simulink library "PRISMA"  (R2025b)
settings: Solver=VariableStepAuto  StartTime=0.0  StopTime=10.0  RelTol=1e-3
libraries: $bdroot x116, etargetslib x30, simulink x9
(part 3 of 3)

== system PRISMA/Transformation/Transform Quaternion OpenGL to NED ==
  OpenGL : Inport  OutDataTypeStr=double  PortDimensions=4
  Mux : Mux
  Selector : Selector  InputPortWidth=4  IndexOptions=Index vector (dialog)  Indices=3  OutputSizes=1
  Selector1 : Selector  InputPortWidth=4  IndexOptions=Index vector (dialog)  Indices=2  OutputSizes=1
  Selector2 : Selector  InputPortWidth=4  IndexOptions=Index vector (dialog)  Indices=4  OutputSizes=1
  Selector3 : Selector  InputPortWidth=4  IndexOptions=Index vector (dialog)  Indices=1  OutputSizes=1
  Unary Minus : UnaryMinus
  Unary Minus1 : UnaryMinus
  NED : Outport  OutDataTypeStr=double  PortDimensions=4
  wires:
  Selector3/1 -> Mux/1
  OpenGL/1 -> Selector/1, Selector1/1, Selector2/1, Selector3/1
  Mux/1 -> NED/1
  Unary Minus/1 -> Mux/2
  Unary Minus1/1 -> Mux/4
  Selector2/1 -> Unary Minus/1
  Selector1/1 -> Mux/3
  Selector/1 -> Unary Minus1/1

== system PRISMA/Transformation/Transform Scale NED to OpenGL ==
  NED : Inport  OutDataTypeStr=double  PortDimensions=3
  Mux : Mux  Inputs=3
  Selector : Selector  InputPortWidth=3  IndexOptions=Index vector (dialog)  Indices=2  OutputSizes=1
  Selector1 : Selector  InputPortWidth=3  IndexOptions=Index vector (dialog)  Indices=1  OutputSizes=1
  Selector2 : Selector  InputPortWidth=3  IndexOptions=Index vector (dialog)  Indices=3  OutputSizes=1
  OpenGL : Outport  OutDataTypeStr=double  PortDimensions=3
  wires:
  Mux/1 -> OpenGL/1
  NED/1 -> Selector2/1, Selector1/1, Selector/1
  Selector2/1 -> Mux/2
  Selector/1 -> Mux/1
  Selector1/1 -> Mux/3

== system PRISMA/Transformation/Transform Scale OpenGL to NED ==
  OpenGL : Inport  OutDataTypeStr=double  PortDimensions=3
  Mux : Mux  Inputs=3
  Selector : Selector  InputPortWidth=3  IndexOptions=Index vector (dialog)  Indices=3  OutputSizes=1
  Selector1 : Selector  InputPortWidth=3  IndexOptions=Index vector (dialog)  Indices=2  OutputSizes=1
  Selector2 : Selector  InputPortWidth=3  IndexOptions=Index vector (dialog)  Indices=1  OutputSizes=1
  NED : Outport  OutDataTypeStr=double  PortDimensions=3
  wires:
  Selector1/1 -> Mux/3
  OpenGL/1 -> Selector2/1, Selector1/1, Selector/1
  Selector2/1 -> Mux/2
  Mux/1 -> NED/1
  Selector/1 -> Mux/1

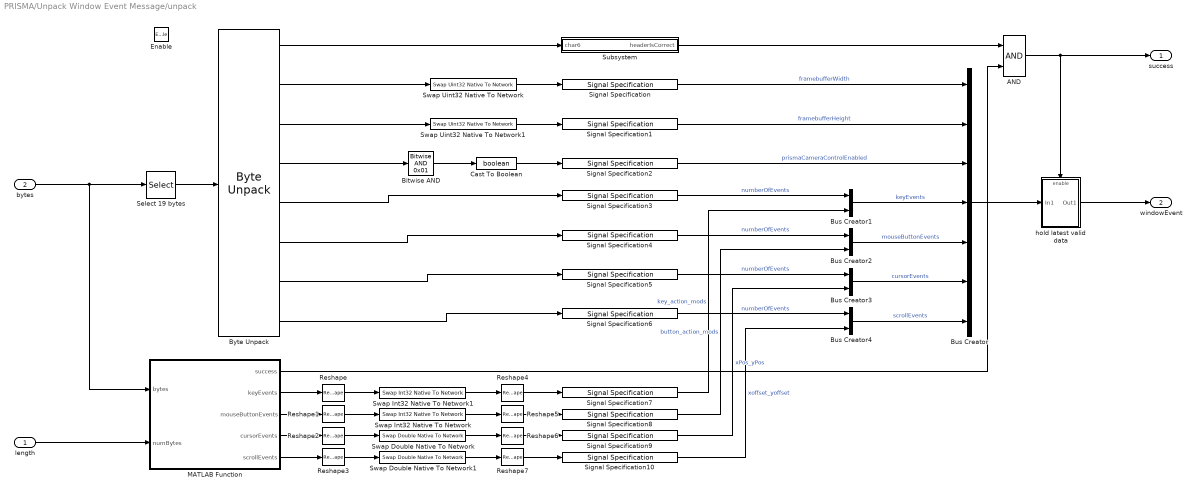
== system PRISMA/Unpack Window Event Message/unpack ==
  length : Inport
  bytes : Inport  Port=2
  Enable : EnablePort
  AND : Logic  AllPortsSameDT=off  OutDataTypeStr=boolean
  Bitwise AND : simulink/Logic and Bit Operations/Bitwise Operator  logicop=AND  UseBitMask=on  BitMask=0x01  BitMaskRealWorld=Stored Integer
      settings: LibrarySourceBlock=|
      | simulink/Quick Insert/Logic and Bit
      | Operations/Bitwise AND
  Bus Creator : BusCreator  Inputs=7
  Bus Creator{1..4} (4 alike) : BusCreator  Inputs=2
  Byte Unpack : etargetslib/Byte Unpack  dimensions={6,1,1,1,1,1,1,1}  datatypes={'uint8','uint32','uint32','uint8','uint8','uint8','uint8','uint8'}  byteAlign=1
      settings: LibrarySourceBlock=embeddedtargetslib/Host Communication/Byte Unpack
  Cast To Boolean : DataTypeConversion  OutDataTypeStr=boolean  SaturateOnIntegerOverflow=off  RndMeth=Floor
  MATLAB Function : MATLAB Function  TreatAsAtomicUnit=on
  Reshape{,1..3} (4 alike) : Reshape
  Reshape4 : Reshape  OutputDimensionality=Customize  OutputDimensions=[255,3]
  Reshape5 : Reshape  OutputDimensionality=Customize  OutputDimensions=[255,3]
  Reshape6 : Reshape  OutputDimensionality=Customize  OutputDimensions=[255,2]
  Reshape7 : Reshape  OutputDimensionality=Customize  OutputDimensions=[255,2]
  Select 19 bytes : Selector  IndexOptions=Index vector (dialog)  Indices=1:19  OutputSizes=1
  Signal Specification : SignalSpecification  OutDataTypeStr=uint32  Dimensions=1
  Signal Specification1 : SignalSpecification  OutDataTypeStr=uint32  Dimensions=1
  Signal Specification10 : SignalSpecification  OutDataTypeStr=double  Dimensions=[255,2]
  Signal Specification2 : SignalSpecification  OutDataTypeStr=boolean  Dimensions=1
  Signal Specification{3..6} (4 alike) : SignalSpecification  OutDataTypeStr=uint8  Dimensions=1
  Signal Specification7 : SignalSpecification  OutDataTypeStr=int32  Dimensions=[255,3]
  Signal Specification8 : SignalSpecification  OutDataTypeStr=int32  Dimensions=[255,3]
  Signal Specification9 : SignalSpecification  OutDataTypeStr=double  Dimensions=[255,2]
  Subsystem : Subsystem
  Swap Double Native To Network : $bdroot/details/Swap Double Native To Network
  Swap Double Native To Network1 : $bdroot/details/Swap Double Native To Network
  Swap Int32 Native To Network : $bdroot/details/Swap Int32 Native To Network
  Swap Int32 Native To Network1 : $bdroot/details/Swap Int32 Native To Network
  Swap Uint32 Native To Network : $bdroot/details/Swap Uint32 Native To Network
  Swap Uint32 Native To Network1 : $bdroot/details/Swap Uint32 Native To Network
  hold latest valid data : Subsystem  TreatAsAtomicUnit=on
  success : Outport  OutDataTypeStr=boolean  PortDimensions=1
  windowEvent : Outport  Port=2
  wires:
  Cast To Boolean/1 -> Signal Specification2/1
  Select 19 bytes/1 -> Byte Unpack/1
  bytes/1 -> Select 19 bytes/1, MATLAB Function/1(bytes)
  Byte Unpack/2 -> Swap Uint32 Native To Network/1
  Byte Unpack/3 -> Swap Uint32 Native To Network1/1
  Byte Unpack/1 -> Subsystem/1(char6)
  Signal Specification/1 -> Bus Creator/1  "framebufferWidth"
  Signal Specification1/1 -> Bus Creator/2  "framebufferHeight"
  Byte Unpack/4 -> Bitwise AND/1
  Bitwise AND/1 -> Cast To Boolean/1
  Byte Unpack/5 -> Signal Specification3/1
  Byte Unpack/6 -> Signal Specification4/1
  Byte Unpack/7 -> Signal Specification5/1
  Byte Unpack/8 -> Signal Specification6/1
  Signal Specification2/1 -> Bus Creator/3  "prismaCameraControlEnabled"
  length/1 -> MATLAB Function/2(numBytes)
  MATLAB Function/2(keyEvents) -> Reshape/1
  MATLAB Function/3(mouseButtonEvents) -> Reshape1/1
  Signal Specification7/1 -> Bus Creator1/2  "key_action_mods"
  Signal Specification8/1 -> Bus Creator2/2  "button_action_mods"
  MATLAB Function/4(cursorEvents) -> Reshape2/1
  MATLAB Function/5(scrollEvents) -> Reshape3/1
  Signal Specification9/1 -> Bus Creator3/2  "xPos_yPos"
  Signal Specification10/1 -> Bus Creator4/2  "xoffset_yoffset"
  Signal Specification3/1 -> Bus Creator1/1  "numberOfEvents"
  Bus Creator1/1 -> Bus Creator/4  "keyEvents"
  Bus Creator2/1 -> Bus Creator/5  "mouseButtonEvents"
  Signal Specification4/1 -> Bus Creator2/1  "numberOfEvents"
  Bus Creator3/1 -> Bus Creator/6  "cursorEvents"
  Signal Specification5/1 -> Bus Creator3/1  "numberOfEvents"
  Bus Creator4/1 -> Bus Creator/7  "scrollEvents"
  Signal Specification6/1 -> Bus Creator4/1  "numberOfEvents"
  Subsystem/1(headerIsCorrect) -> AND/1
  MATLAB Function/1(success) -> AND/2
  AND/1 -> success/1, hold latest valid data/Enable
  Bus Creator/1 -> hold latest valid data/1(In1)
  hold latest valid data/1(Out1) -> windowEvent/1
  Swap Uint32 Native To Network/1 -> Signal Specification/1
  Swap Uint32 Native To Network1/1 -> Signal Specification1/1
  Swap Double Native To Network/1 -> Reshape6/1
  Swap Double Native To Network1/1 -> Reshape7/1
  Swap Int32 Native To Network/1 -> Reshape5/1
  Swap Int32 Native To Network1/1 -> Reshape4/1
  Reshape/1 -> Swap Int32 Native To Network1/1
  Reshape1/1 -> Swap Int32 Native To Network/1
  Reshape2/1 -> Swap Double Native To Network/1
  Reshape3/1 -> Swap Double Native To Network1/1
  Reshape4/1 -> Signal Specification7/1
  Reshape5/1 -> Signal Specification8/1
  Reshape6/1 -> Signal Specification9/1
  Reshape7/1 -> Signal Specification10/1

== system PRISMA/details/PRISMA Bitfield To Byte ==
  bitfield : Inport  OutDataTypeStr=boolean  PortDimensions=8
  Bitwise Operator : simulink/Logic and Bit Operations/Bitwise Operator  logicop=OR  UseBitMask=off  NumInputPorts=8  BitMask=bin2dec('11011001')  BitMaskRealWorld=Stored Integer
  Data Type Conversion : DataTypeConversion  OutDataTypeStr=uint8  SaturateOnIntegerOverflow=off  RndMeth=Floor
  Demux6 : Demux  Outputs=8
  Shift Arithmetic : ArithShift  BitShiftNumber=1  BitShiftDirection=Left
  Shift Arithmetic1 : ArithShift  BitShiftNumber=2  BitShiftDirection=Left
  Shift Arithmetic2 : ArithShift  BitShiftNumber=3  BitShiftDirection=Left
  Shift Arithmetic3 : ArithShift  BitShiftNumber=4  BitShiftDirection=Left
  Shift Arithmetic4 : ArithShift  BitShiftNumber=5  BitShiftDirection=Left
  Shift Arithmetic5 : ArithShift  BitShiftNumber=6  BitShiftDirection=Left
  Shift Arithmetic6 : ArithShift  BitShiftNumber=7  BitShiftDirection=Left
  byte : Outport  OutDataTypeStr=uint8  PortDimensions=1
  wires:
  Demux6/4 -> Shift Arithmetic2/1
  Demux6/5 -> Shift Arithmetic3/1
  Data Type Conversion/1 -> Demux6/1
  Demux6/2 -> Shift Arithmetic/1
  Shift Arithmetic1/1 -> Bitwise Operator/3
  Demux6/7 -> Shift Arithmetic5/1
  Demux6/6 -> Shift Arithmetic4/1
  Shift Arithmetic6/1 -> Bitwise Operator/8
  Shift Arithmetic5/1 -> Bitwise Operator/7
  Shift Arithmetic/1 -> Bitwise Operator/2
  Demux6/1 -> Bitwise Operator/1
  Demux6/3 -> Shift Arithmetic1/1
  Shift Arithmetic4/1 -> Bitwise Operator/6
  Demux6/8 -> Shift Arithmetic6/1
  Bitwise Operator/1 -> byte/1
  Shift Arithmetic3/1 -> Bitwise Operator/5
  Shift Arithmetic2/1 -> Bitwise Operator/4
  bitfield/1 -> Data Type Conversion/1

== system PRISMA/details/PRISMA Message Type ==
  value : Constant  Value=messageType - 1  OutDataTypeStr=uint8
  byte : Outport  OutDataTypeStr=uint8  PortDimensions=1
  wires:
  value/1 -> byte/1

== system PRISMA/details/Swap Double Native To Network ==
  note: Check endianess of this machine
      | (only swap on little-endian-based machines)
  in : Inport  OutDataTypeStr=double
  Byte Pack1 : etargetslib/Byte Pack  datatypes={'uint16'}  byteAlign=1
  Constant : Constant  Value=uint16(1)
  Selector2 : Selector  InputPortWidth=2  IndexOptions=Index vector (dialog)  Indices=1  OutputSizes=1
  Swap Each Element : Subsystem  TreatAsAtomicUnit=on
  Switch : Switch  Criteria=u2 ~= 0  SaturateOnIntegerOverflow=off  InputSameDT=off
  out : Outport  OutDataTypeStr=double
  wires:
  Switch/1 -> out/1
  Selector2/1 -> Switch/2
  Swap Each Element/1(out) -> Switch/1
  Byte Pack1/1 -> Selector2/1
  in/1 -> Swap Each Element/1(in), Switch/3
  Constant/1 -> Byte Pack1/1

== system PRISMA/details/Swap Float Native To Network ==
  note: Check endianess of this machine
      | (only swap on little-endian-based machines)
  in : Inport  OutDataTypeStr=single
  Byte Pack1 : etargetslib/Byte Pack  datatypes={'uint16'}  byteAlign=1
  Constant : Constant  Value=uint16(1)
  Selector2 : Selector  InputPortWidth=2  IndexOptions=Index vector (dialog)  Indices=1  OutputSizes=1
  Swap Each Element : Subsystem  TreatAsAtomicUnit=on
  Switch : Switch  Criteria=u2 ~= 0  SaturateOnIntegerOverflow=off  InputSameDT=off
  out : Outport  OutDataTypeStr=single
  wires:
  Constant/1 -> Byte Pack1/1
  in/1 -> Switch/3, Swap Each Element/1(in)
  Byte Pack1/1 -> Selector2/1
  Swap Each Element/1(out) -> Switch/1
  Selector2/1 -> Switch/2
  Switch/1 -> out/1

== system PRISMA/details/Swap Int32 Native To Network ==
  note: Check endianess of this machine
      | (only swap on little-endian-based machines)
  in : Inport  OutDataTypeStr=int32
  Byte Pack1 : etargetslib/Byte Pack  datatypes={'uint16'}  byteAlign=1
  Constant : Constant  Value=uint16(1)
  Selector2 : Selector  InputPortWidth=2  IndexOptions=Index vector (dialog)  Indices=1  OutputSizes=1
  Swap Each Element : Subsystem  TreatAsAtomicUnit=on
  Switch : Switch  Criteria=u2 ~= 0  SaturateOnIntegerOverflow=off  InputSameDT=off
  out : Outport  OutDataTypeStr=int32
  wires:
  Constant/1 -> Byte Pack1/1
  in/1 -> Switch/3, Swap Each Element/1(in)
  Byte Pack1/1 -> Selector2/1
  Swap Each Element/1(out) -> Switch/1
  Selector2/1 -> Switch/2
  Switch/1 -> out/1

== system PRISMA/details/Swap Uint16 Native To Network ==
  note: Check endianess of this machine
      | (only swap on little-endian-based machines)
  in : Inport  OutDataTypeStr=uint16
  Byte Pack1 : etargetslib/Byte Pack  datatypes={'uint16'}  byteAlign=1
  Constant : Constant  Value=uint16(1)
  Selector2 : Selector  InputPortWidth=2  IndexOptions=Index vector (dialog)  Indices=1  OutputSizes=1
  Swap Each Element : Subsystem  TreatAsAtomicUnit=on
  Switch : Switch  Criteria=u2 ~= 0  SaturateOnIntegerOverflow=off  InputSameDT=off
  out : Outport  OutDataTypeStr=uint16
  wires:
  Switch/1 -> out/1
  Selector2/1 -> Switch/2
  Swap Each Element/1(out) -> Switch/1
  Byte Pack1/1 -> Selector2/1
  in/1 -> Swap Each Element/1(in), Switch/3
  Constant/1 -> Byte Pack1/1

== system PRISMA/details/Swap Uint32 Native To Network ==
  note: Check endianess of this machine
      | (only swap on little-endian-based machines)
  in : Inport  OutDataTypeStr=uint32
  Byte Pack1 : etargetslib/Byte Pack  datatypes={'uint16'}  byteAlign=1
  Constant : Constant  Value=uint16(1)
  Selector2 : Selector  InputPortWidth=2  IndexOptions=Index vector (dialog)  Indices=1  OutputSizes=1
  Swap Each Element : Subsystem  TreatAsAtomicUnit=on
  Switch : Switch  Criteria=u2 ~= 0  SaturateOnIntegerOverflow=off  InputSameDT=off
  out : Outport  OutDataTypeStr=uint32
  wires:
  Switch/1 -> out/1
  Selector2/1 -> Switch/2
  Swap Each Element/1(out) -> Switch/1
  Byte Pack1/1 -> Selector2/1
  in/1 -> Swap Each Element/1(in), Switch/3
  Constant/1 -> Byte Pack1/1

== system PRISMA/Unpack Window Event Message/unpack/Subsystem ==
  char6 : Inport
  AND : Logic  Inputs=6  AllPortsSameDT=off  OutDataTypeStr=boolean
  Compare To Constant : simulink/Logic and Bit Operations/Compare To Constant  relop===  const=uint8('P')  OutDataTypeStr=boolean
  Compare To Constant1 : simulink/Logic and Bit Operations/Compare To Constant  relop===  const=uint8('R')  OutDataTypeStr=boolean
  Compare To Constant2 : simulink/Logic and Bit Operations/Compare To Constant  relop===  const=uint8('I')  OutDataTypeStr=boolean
  Compare To Constant3 : simulink/Logic and Bit Operations/Compare To Constant  relop===  const=uint8('S')  OutDataTypeStr=boolean
  Compare To Constant4 : simulink/Logic and Bit Operations/Compare To Constant  relop===  const=uint8('M')  OutDataTypeStr=boolean
  Compare To Constant5 : simulink/Logic and Bit Operations/Compare To Constant  relop===  const=uint8('A')  OutDataTypeStr=boolean
  Demux : Demux  Outputs=6
  headerIsCorrect : Outport
  wires:
  Demux/5 -> Compare To Constant4/1
  Compare To Constant1/1 -> AND/2
  Compare To Constant2/1 -> AND/3
  Demux/2 -> Compare To Constant1/1
  Compare To Constant5/1 -> AND/6
  Demux/1 -> Compare To Constant/1
  Demux/3 -> Compare To Constant2/1
  Demux/4 -> Compare To Constant3/1
  Compare To Constant3/1 -> AND/4
  Compare To Constant/1 -> AND/1
  Compare To Constant4/1 -> AND/5
  Demux/6 -> Compare To Constant5/1
  AND/1 -> headerIsCorrect/1
  char6/1 -> Demux/1

== system PRISMA/Unpack Window Event Message/unpack/hold latest valid data ==
  In1 : Inport
  Enable : EnablePort
  Out1 : Outport
  wires:
  In1/1 -> Out1/1

== system PRISMA/details/Swap Double Native To Network/Swap Each Element ==
  in : Inport  Partition=on  PartitionDimension=1  PartitionWidth=1  PartitionOffset=0
  Byte Pack : etargetslib/Byte Pack  datatypes={'double'}  byteAlign=1
  Byte Unpack : etargetslib/Byte Unpack  dimensions={[1]}  datatypes={'double'}  byteAlign=1
  For Each : ForEach  DisableCoverage=on
  Selector : Selector  InputPortWidth=8  IndexOptions=Index vector (dialog)  Indices=[8 7 6 5 4 3 2 1]  OutputSizes=1
  out : Outport  ConcatenationDimension=1
  wires:
  in/1 -> Byte Pack/1
  Byte Unpack/1 -> out/1
  Byte Pack/1 -> Selector/1
  Selector/1 -> Byte Unpack/1

== system PRISMA/details/Swap Float Native To Network/Swap Each Element ==
  in : Inport  Partition=on  PartitionDimension=1  PartitionWidth=1  PartitionOffset=0
  Byte Pack : etargetslib/Byte Pack  datatypes={'single'}  byteAlign=1
  Byte Unpack : etargetslib/Byte Unpack  dimensions={[1]}  datatypes={'single'}  byteAlign=1
  For Each : ForEach  DisableCoverage=on
  Selector : Selector  InputPortWidth=4  IndexOptions=Index vector (dialog)  Indices=[4 3 2 1]  OutputSizes=1
  out : Outport  ConcatenationDimension=1
  wires:
  Selector/1 -> Byte Unpack/1
  Byte Pack/1 -> Selector/1
  Byte Unpack/1 -> out/1
  in/1 -> Byte Pack/1

== system PRISMA/details/Swap Int32 Native To Network/Swap Each Element ==
  in : Inport  Partition=on  PartitionDimension=1  PartitionWidth=1  PartitionOffset=0
  Byte Pack : etargetslib/Byte Pack  datatypes={'int32'}  byteAlign=1
  Byte Unpack : etargetslib/Byte Unpack  dimensions={[1]}  datatypes={'int32'}  byteAlign=1
  For Each : ForEach  DisableCoverage=on
  Selector : Selector  InputPortWidth=4  IndexOptions=Index vector (dialog)  Indices=[4 3 2 1]  OutputSizes=1
  out : Outport  ConcatenationDimension=1
  wires:
  Selector/1 -> Byte Unpack/1
  Byte Pack/1 -> Selector/1
  Byte Unpack/1 -> out/1
  in/1 -> Byte Pack/1

== system PRISMA/details/Swap Uint16 Native To Network/Swap Each Element ==
  in : Inport  Partition=on  PartitionDimension=1  PartitionWidth=1  PartitionOffset=0
  Byte Pack : etargetslib/Byte Pack  datatypes={'uint16'}  byteAlign=1
  Byte Unpack : etargetslib/Byte Unpack  dimensions={[1]}  datatypes={'uint16'}  byteAlign=1
  For Each : ForEach  DisableCoverage=on
  Selector : Selector  InputPortWidth=2  IndexOptions=Index vector (dialog)  Indices=[2 1]  OutputSizes=1
  out : Outport  ConcatenationDimension=1
  wires:
  in/1 -> Byte Pack/1
  Byte Unpack/1 -> out/1
  Byte Pack/1 -> Selector/1
  Selector/1 -> Byte Unpack/1

== system PRISMA/details/Swap Uint32 Native To Network/Swap Each Element ==
  in : Inport  Partition=on  PartitionDimension=1  PartitionWidth=1  PartitionOffset=0
  Byte Pack : etargetslib/Byte Pack  datatypes={'uint32'}  byteAlign=1
  Byte Unpack : etargetslib/Byte Unpack  dimensions={[1]}  datatypes={'uint32'}  byteAlign=1
  For Each : ForEach  DisableCoverage=on
  Selector : Selector  InputPortWidth=4  IndexOptions=Index vector (dialog)  Indices=[4 3 2 1]  OutputSizes=1
  out : Outport  ConcatenationDimension=1
  wires:
  in/1 -> Byte Pack/1
  Byte Unpack/1 -> out/1
  Byte Pack/1 -> Selector/1
  Selector/1 -> Byte Unpack/1

== matlab function PRISMA/Transformation/Euler ZYX to Quaternion/MATLAB Function ==
  data: roll input; q output; pitch input; yaw input
function q = EulerToQuaternionZYX(roll, pitch, yaw)
    q = eul2quat([yaw, pitch, roll],'ZYX')';
end

== matlab function PRISMA/Pack Watermesh Message/Serialize To Network Byte Order ==
  data: vertexData input single size=[2,255,32]; bytes output uint8 size=65280; numVertices input uint8 size=32; numPolygons input uint8 size=1; numBytes output int32 size=1
function [bytes, numBytes] = SerializeWatermeshData(vertexData, numVertices, numPolygons)
    tmp = typecast(uint16(1),'uint8');
    swapByteOrder = (tmp(1) == uint8(1));

    % output size
    bytes = uint8(zeros(65280,1)); % 2*255*32 * 4
    numBytes = int32(0);

    % number of polygons (2 bytes)
    numPolygons = uint16(min(uint16(numPolygons), uint16(32)));
    bytes(1:2) = reshape(typecast(uint16(numPolygons),'uint8'), [2 1]);
    if(swapByteOrder)
        h = bytes(1);
        bytes(1) = bytes(2);
        bytes(2) = h;
    end

    % serialize all polygons
    index = int32(3);
    if(swapByteOrder)
        for p = uint32(1):uint32(numPolygons)
            % number of vertices (2 bytes)
            N = uint16(numVertices(p));
            bytes(index:(index+int32(1))) = reshape(typecast(uint16(N),'uint8'), [2 1]);
            h = bytes(index);
            bytes(index) = bytes(index+int32(1));
            bytes(index+int32(1)) = h;
            index = index + int32(2);
    
            % serialize all vertices
            for n = uint32(1):uint32(N)
                x = single(vertexData(1,n,p));
                y = single(vertexData(2,n,p));
                bytes(index:(index+int32(3))) = reshape(typecast(single(x),'uint8'), [4 1]);
                h = bytes(index);
                bytes(index) = bytes(index+int32(3));
                bytes(index+int32(3)) = h;
                h = bytes(index+int32(1));
                bytes(index+int32(1)) = bytes(index+int32(2));
                bytes(index+int32(2)) = h;
                index = index + int32(4);
                bytes(index:(index+int32(3))) = reshape(typecast(single(y),'uint8'), [4 1]);
                h = bytes(index);
                bytes(index) = bytes(index+int32(3));
                bytes(index+int32(3)) = h;
                h = bytes(index+int32(1));
                bytes(index+int32(1)) = bytes(index+int32(2));
                bytes(index+int32(2)) = h;
                index = index + int32(4);
            end
        end
    else
        for p = uint32(1):uint32(numPolygons)
            % number of vertices (2 bytes)
            N = uint16(numVertices(p));
            bytes(index:(index+int32(1))) = reshape(typecast(uint16(N),'uint8'), [2 1]);
            index = index + int32(2);
    
            % serialize all vertices
            for n = uint32(1):uint32(N)
                x = single(vertexData(1,n,p));
                y = single(vertexData(2,n,p));
                bytes(index:(index+int32(3))) = reshape(typecast(single(x),'uint8'), [4 1]);
                index = index + int32(4);
                bytes(index:(index+int32(3))) = reshape(typecast(single(y),'uint8'), [4 1]);
                index = index + int32(4);
            end
        end
    end

    % number of bytes
    numBytes = index - int32(1);
end

== matlab function PRISMA/Transformation/Look At to Quaternion/MATLAB Function ==
  data: eyePosition input; quaternion output; lookAtPosition input
function quaternion = Wrapper_LookAtToQuaternion(eyePosition, lookAtPosition)
    quaternion = PRISMA.LookAtToQuaternion(eyePosition, lookAtPosition);
end

== matlab function PRISMA/Transformation/Quaternion to Rotation Matrix/MATLAB Function ==
  data: q input; dcm output
function dcm = QuaternionToRM(q)
    dcm = quat2rotm([q(1), q(2), q(3), q(4)]);
end

== matlab function PRISMA/Pack Dynamic Mesh Message/Serialize To Network Byte Order ==
  data: vertexData input single size=[6,2000]; bytes output uint8 size=65411; numVertices input uint16 size=1; indexData input uint16 size=10000; numBytes output int32 size=1; numIndices input uint16 size=1
function [bytes, numBytes] = SerializeDynamicMeshData(vertexData, numVertices, indexData, numIndices)
    tmp = typecast(uint16(1),'uint8');
    swapByteOrder = (tmp(1) == uint8(1));

    % output size
    bytes = uint8(zeros(65411,1)); % 65507-92-4
    numBytes = int32(0);

    % number of vertices (2 bytes)
    numVertices = uint16(min(uint16(numVertices), uint16(2000)));
    bytes(1:2) = reshape(typecast(uint16(numVertices),'uint8'), [2 1]);
    if(swapByteOrder)
        h = bytes(1);
        bytes(1) = bytes(2);
        bytes(2) = h;
    end

    % serialize all vertices
    index = int32(3);
    if(swapByteOrder)
        for n = uint32(1):uint32(numVertices)
            bytes(index:(index+int32(3))) = reshape(typecast(single(vertexData(1,n)),'uint8'), [4 1]);    h = bytes(index); bytes(index) = bytes(index+int32(3)); bytes(index+int32(3)) = h; h = bytes(index+int32(1)); bytes(index+1) = bytes(index+int32(2)); bytes(index+int32(2)) = h;    index = index + int32(4);
            bytes(index:(index+int32(3))) = reshape(typecast(single(vertexData(2,n)),'uint8'), [4 1]);    h = bytes(index); bytes(index) = bytes(index+int32(3)); bytes(index+int32(3)) = h; h = bytes(index+int32(1)); bytes(index+1) = bytes(index+int32(2)); bytes(index+int32(2)) = h;    index = index + int32(4);
            bytes(index:(index+int32(3))) = reshape(typecast(single(vertexData(3,n)),'uint8'), [4 1]);    h = bytes(index); bytes(index) = bytes(index+int32(3)); bytes(index+int32(3)) = h; h = bytes(index+int32(1)); bytes(index+1) = bytes(index+int32(2)); bytes(index+int32(2)) = h;    index = index + int32(4);
            bytes(index:(index+int32(3))) = reshape(typecast(single(vertexData(4,n)),'uint8'), [4 1]);    h = bytes(index); bytes(index) = bytes(index+int32(3)); bytes(index+int32(3)) = h; h = bytes(index+int32(1)); bytes(index+1) = bytes(index+int32(2)); bytes(index+int32(2)) = h;    index = index + int32(4);
            bytes(index:(index+int32(3))) = reshape(typecast(single(vertexData(5,n)),'uint8'), [4 1]);    h = bytes(index); bytes(index) = bytes(index+int32(3)); bytes(index+int32(3)) = h; h = bytes(index+int32(1)); bytes(index+1) = bytes(index+int32(2)); bytes(index+int32(2)) = h;    index = index + int32(4);
            bytes(index:(index+int32(3))) = reshape(typecast(single(vertexData(6,n)),'uint8'), [4 1]);    h = bytes(index); bytes(index) = bytes(index+int32(3)); bytes(index+int32(3)) = h; h = bytes(index+int32(1)); bytes(index+1) = bytes(index+int32(2)); bytes(index+int32(2)) = h;    index = index + int32(4);
        end
    else
        for n = uint32(1):uint32(numVertices)
            bytes(index:(index+int32(3))) = reshape(typecast(single(vertexData(1,n)),'uint8'), [4 1]);    index = index + int32(4);
            bytes(index:(index+int32(3))) = reshape(typecast(single(vertexData(2,n)),'uint8'), [4 1]);    index = index + int32(4);
            bytes(index:(index+int32(3))) = reshape(typecast(single(vertexData(3,n)),'uint8'), [4 1]);    index = index + int32(4);
            bytes(index:(index+int32(3))) = reshape(typecast(single(vertexData(4,n)),'uint8'), [4 1]);    index = index + int32(4);
            bytes(index:(index+int32(3))) = reshape(typecast(single(vertexData(5,n)),'uint8'), [4 1]);    index = index + int32(4);
            bytes(index:(index+int32(3))) = reshape(typecast(single(vertexData(6,n)),'uint8'), [4 1]);    index = index + int32(4);
        end
    end

    % number of indices (2 bytes)
    numIndices = uint16(min(uint16(numIndices), uint16(10000)));
    bytes(index:(index+int32(1))) = reshape(typecast(uint16(numIndices),'uint8'), [2 1]);
    if(swapByteOrder)
        h = bytes(index);
        bytes(index) = bytes(index+int32(1));
        bytes(index+int32(1)) = h;
    end
    index = index + int32(2);

    % serialize all indices
    if(swapByteOrder)
        for n = uint32(1):uint32(numIndices)
            bytes(index:(index+int32(1))) = reshape(typecast(uint16(indexData(n)),'uint8'), [2 1]);    h = bytes(index); bytes(index) = bytes(index+int32(1)); bytes(index+int32(1)) = h;    index = index + int32(2);
        end
    else
        for n = uint32(1):uint32(numIndices)
            bytes(index:(index+int32(1))) = reshape(typecast(uint16(indexData(n)),'uint8'), [2 1]);    index = index + int32(2);
        end
    end

    % number of bytes
    numBytes = index - int32(1);
end

== matlab function PRISMA/Unpack Window Event Message/unpack/MATLAB Function ==
  data: bytes input uint8; success output boolean size=1; numBytes input int32 size=1; keyEvents output int32 size=[255 3]; mouseButtonEvents output int32 size=[255 3]; cursorEvents output double size=[255 2]; scrollEvents output double size=[255 2]
function [success, keyEvents, mouseButtonEvents, cursorEvents, scrollEvents] = UnpackVariableLengthData(bytes, numBytes)
    % set default output
    success = false;
    keyEvents = int32(zeros(255,3));
    mouseButtonEvents = int32(zeros(255,3));
    cursorEvents = double(zeros(255,2));
    scrollEvents = double(zeros(255,2));

    % check for correct message size
    numKeyEvents = uint32(bytes(16));
    numMouseButtonEvents = uint32(bytes(17));
    numCursorEvents = uint32(bytes(18));
    numScrollEvents = uint32(bytes(19));
    if(numBytes ~= (int32(19) + int32(numKeyEvents + numMouseButtonEvents)*int32(12) + int32(numCursorEvents + numScrollEvents)*int32(16)))
        return;
    end

    % unpack all events
    i = uint32(20); % one-based index
    for n = uint32(1):numKeyEvents
        keyEvents(n,1) = int32(typecast(uint8(bytes(i:(i+uint32(3)))), 'int32'));    i = i + uint32(4);
        keyEvents(n,2) = int32(typecast(uint8(bytes(i:(i+uint32(3)))), 'int32'));    i = i + uint32(4);
        keyEvents(n,3) = int32(typecast(uint8(bytes(i:(i+uint32(3)))), 'int32'));    i = i + uint32(4);
    end
    for n = uint32(1):numMouseButtonEvents
        mouseButtonEvents(n,1) = int32(typecast(uint8(bytes(i:(i+uint32(3)))), 'int32'));    i = i + uint32(4);
        mouseButtonEvents(n,2) = int32(typecast(uint8(bytes(i:(i+uint32(3)))), 'int32'));    i = i + uint32(4);
        mouseButtonEvents(n,3) = int32(typecast(uint8(bytes(i:(i+uint32(3)))), 'int32'));    i = i + uint32(4);
    end
    for n = uint32(1):numCursorEvents
        cursorEvents(n,1) = double(typecast(uint8(bytes(i:(i+uint32(7)))), 'double'));    i = i + uint32(8);
        cursorEvents(n,2) = double(typecast(uint8(bytes(i:(i+uint32(7)))), 'double'));    i = i + uint32(8);
    end
    for n = uint32(1):numScrollEvents
        scrollEvents(n,1) = double(typecast(uint8(bytes(i:(i+uint32(7)))), 'double'));    i = i + uint32(8);
        scrollEvents(n,2) = double(typecast(uint8(bytes(i:(i+uint32(7)))), 'double'));    i = i + uint32(8);
    end
    success = true;
end

== matlab function PRISMA/Sun Light Color/MATLAB Function1 ==
  data: eyePosition input double size=3; lightColor output double size=3; sunLightDirection input double size=3; radiusPlanet input double size=1; radiusAtmosphere input double size=1; scaleHeightRayleigh input double size=1; coefficientRayleigh input double size=3; sunIntensity input double size=1
function lightColor = Wrapper_SunLightColor(eyePosition, sunLightDirection, radiusPlanet, radiusAtmosphere, scaleHeightRayleigh, coefficientRayleigh, sunIntensity)
    lightColor = PRISMA.SunLightColor(eyePosition, sunLightDirection, radiusPlanet, radiusAtmosphere, scaleHeightRayleigh, coefficientRayleigh, sunIntensity);
end
